simulink model "modelo"  (R2019b)
settings: Solver=ode45  StartTime=0.0  StopTime=0.5  MaxStep=1e-4  RelTol=1e-3
undefined symbols (not defined in the file or in its folder): GL, HL
settings Model: Creator=l54  LastModifiedBy=B13

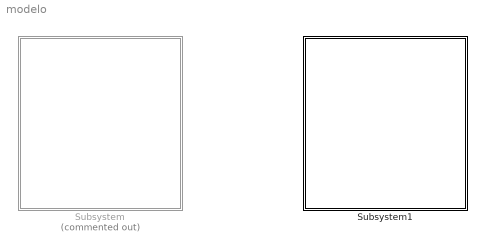
== system modelo ==
  Subsystem : Subsystem  Commented=on
  Subsystem1 : Subsystem

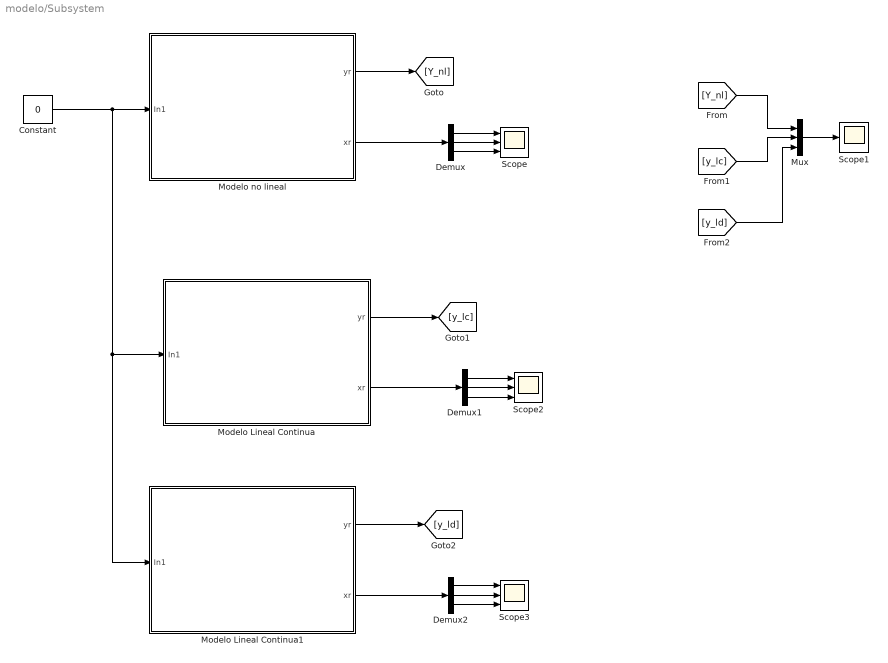
== system modelo/Subsystem ==
  Constant : Constant  Value=0
  Demux : Demux  Outputs=3
  Demux1 : Demux  Outputs=3
  Demux2 : Demux  Outputs=3
  Modelo Lineal Continua : Subsystem  mask(LEVITADOR MAGNETICO){g=9.81, M=0.05, R=10, L=0.5, xini=[0.01;0;0]}
      mask prompts: g "Gravedad"; M "Masa"; R "Resistencia"; L "Inductancia"; xini "Condiciones Iniciales"
      mask help: MODELO NO LINEAL DE UN LEVITADOR MAGENTICO
      mask init:
      | x10 = 0.16;
      | x20 = 0;
      | x30 = sqrt(g*M*x10);
      | AL = [0, 1, 0;
      |     x30^2/(M*x10^2), 0, -2*x30/(M*x10);
      |     0, 0, -R/L];
      | BL = [0;
      |     0;
      |     1/L];
      | CL = [1 0 0];
      | DL = 0;
      | eo = R*x30;
  Modelo Lineal Continua1 : Subsystem  mask(LEVITADOR MAGNETICO){g=9.81, M=0.05, R=10, L=0.5, xini=[0.01;0;0], Tm=0.01}
      mask prompts: g "Gravedad"; M "Masa"; R "Resistencia"; L "Inductancia"; xini "Condiciones Iniciales"; Tm "Periodo de muestreo"
      mask help: MODELO NO LINEAL DE UN LEVITADOR MAGENTICO
      mask init:
      | x10 = 0.16;
      | x20 = 0;
      | x30 = sqrt(g*M*x10);
      | AL = [0, 1, 0;
      |     x30^2/(M*x10^2), 0, -2*x30/(M*x10);
      |     0, 0, -R/L];
      | BL = [0;
      |     0;
      |     1/L];
      | CL = [1 0 0];
      | DL = 0;
      | eo = R*x30;
      | [GL,HL] = c2d(AL,BL,Tm);
  Modelo no lineal : Subsystem  mask(LEVITADOR MAGNETICO){g=9.81, M=0.05, R=10, L=0.5, xini=[0.01;0;0]}
      mask prompts: g "Gravedad"; M "Masa"; R "Resistencia"; L "Inductancia"; xini "Condiciones Iniciales"
      mask help: MODELO NO LINEAL DE UN LEVITADOR MAGENTICO
      mask init:
      | x10 = 0.16;
      | x20 = 0;
      | x30 = sqrt(g*M*x10);
      | CL = [1 0 0];
      | DL = 0;
      | eo = R*x30;
  Mux : Mux  Inputs=3
  Scope : Scope  NumInputPorts=3
  Scope1 : Scope
  Scope2 : Scope  NumInputPorts=3
  Scope3 : Scope  NumInputPorts=3
  wires:
  Demux2/3 -> Scope3/3
  [y_ld] -> Mux/3
  Constant/1 -> Modelo Lineal Continua1/1(In1), Modelo Lineal Continua/1(In1), Modelo no lineal/1(In1)
  Mux/1 -> Scope1/1
  Modelo no lineal/1(yr) -> [Y_nl]
  Demux1/3 -> Scope2/3
  Demux2/2 -> Scope3/2
  Demux/3 -> Scope/3
  Demux1/2 -> Scope2/2
  [Y_nl] -> Mux/1
  Demux1/1 -> Scope2/1
  Modelo Lineal Continua1/2(xr) -> Demux2/1
  Modelo Lineal Continua/2(xr) -> Demux1/1
  [y_lc] -> Mux/2
  Demux/2 -> Scope/2
  Modelo Lineal Continua1/1(yr) -> [y_ld]
  Demux/1 -> Scope/1
  Modelo Lineal Continua/1(yr) -> [y_lc]
  Demux2/1 -> Scope3/1
  Modelo no lineal/2(xr) -> Demux/1

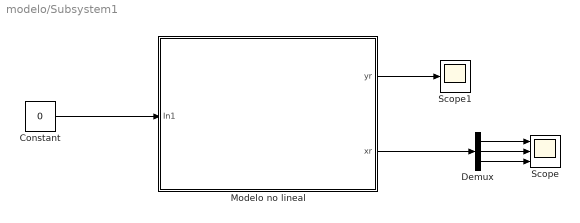
== system modelo/Subsystem1 ==
  Constant : Constant  Value=0
  Demux : Demux  Outputs=3
  Modelo no lineal : Subsystem  mask(LEVITADOR MAGNETICO){g=9.81, M=0.05, R=10, L=0.5, xini=[0;0;0]}
      mask prompts: g "Gravedad"; M "Masa"; R "Resistencia"; L "Inductancia"; xini "Condiciones Iniciales"
      mask help: MODELO NO LINEAL DE UN LEVITADOR MAGENTICO
      mask init:
      | x10 = 0.16;
      | x20 = 0;
      | x30 = sqrt(g*M*x10);
      | CL = [1 0 0];
      | DL = 0;
      | eo = R*x30;
  Scope : Scope  NumInputPorts=3
  Scope1 : Scope
  wires:
  Constant/1 -> Modelo no lineal/1(In1)
  Modelo no lineal/1(yr) -> Scope1/1
  Demux/3 -> Scope/3
  Demux/2 -> Scope/2
  Demux/1 -> Scope/1
  Modelo no lineal/2(xr) -> Demux/1

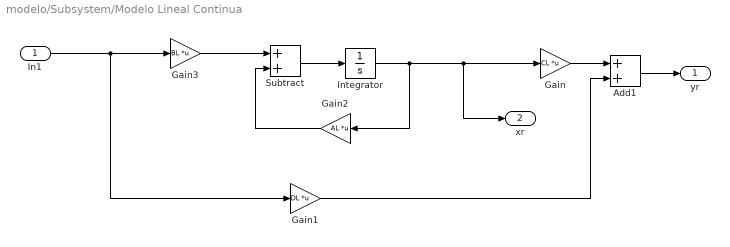
== system modelo/Subsystem/Modelo Lineal Continua ==
  In1 : Inport
  Add1 : Sum
  Gain : Gain  Gain=CL  Multiplication=Matrix(K*u)
  Gain1 : Gain  Gain=DL  Multiplication=Matrix(K*u)
  Gain2 : Gain  Gain=AL  Multiplication=Matrix(K*u)
  Gain3 : Gain  Gain=BL  Multiplication=Matrix(K*u)
  Integrator : Integrator  InitialCondition=xini
  Subtract : Sum
  yr : Outport
  xr : Outport  Port=2
  wires:
  In1/1 -> Gain3/1, Gain1/1
  Integrator/1 -> Gain/1, xr/1, Gain2/1
  Add1/1 -> yr/1
  Gain/1 -> Add1/1
  Gain1/1 -> Add1/2
  Subtract/1 -> Integrator/1
  Gain2/1 -> Subtract/2
  Gain3/1 -> Subtract/1

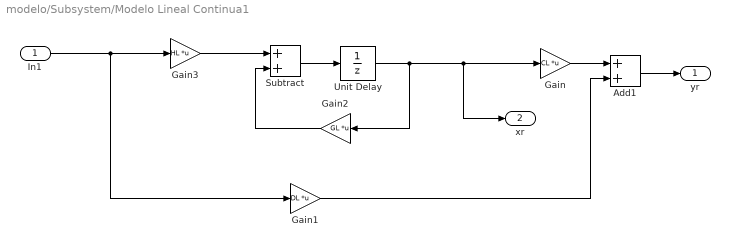
== system modelo/Subsystem/Modelo Lineal Continua1 ==
  In1 : Inport
  Add1 : Sum
  Gain : Gain  Gain=CL  Multiplication=Matrix(K*u)
  Gain1 : Gain  Gain=DL  Multiplication=Matrix(K*u)
  Gain2 : Gain  Gain=GL  Multiplication=Matrix(K*u)
  Gain3 : Gain  Gain=HL  Multiplication=Matrix(K*u)
  Subtract : Sum
  Unit Delay : UnitDelay  InitialCondition=xini  SampleTime=Tm  HasFrameUpgradeWarning=on
  yr : Outport
  xr : Outport  Port=2
  wires:
  In1/1 -> Gain3/1, Gain1/1
  Unit Delay/1 -> Gain/1, xr/1, Gain2/1
  Add1/1 -> yr/1
  Gain/1 -> Add1/1
  Gain1/1 -> Add1/2
  Subtract/1 -> Unit Delay/1
  Gain2/1 -> Subtract/2
  Gain3/1 -> Subtract/1

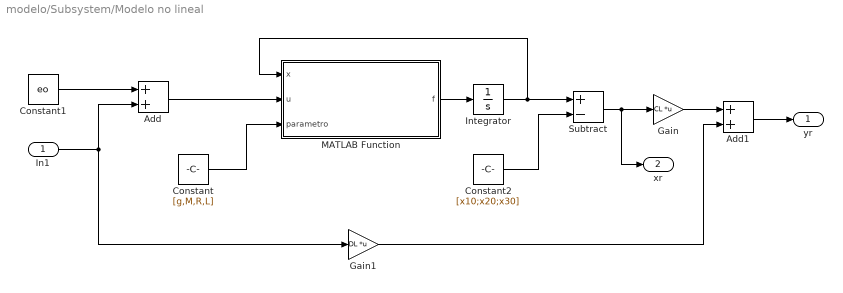
== system modelo/Subsystem/Modelo no lineal ==
  In1 : Inport
  Add : Sum
  Add1 : Sum
  Constant : Constant  Value=[g,M,R,L]
  Constant1 : Constant  Value=eo
  Constant2 : Constant  Value=[x10;x20;x30]
  Gain : Gain  Gain=CL  Multiplication=Matrix(K*u)
  Gain1 : Gain  Gain=DL  Multiplication=Matrix(K*u)
  Integrator : Integrator  InitialCondition=[x10; x20; x30]+xini
  MATLAB Function : MATLAB Function  TreatAsAtomicUnit=on
  Subtract : Sum  Inputs=+-
  yr : Outport
  xr : Outport  Port=2
  wires:
  Integrator/1 -> MATLAB Function/1(x), Subtract/1
  In1/1 -> Gain1/1, Add/2
  MATLAB Function/1(f) -> Integrator/1
  Add/1 -> MATLAB Function/2(u)
  Constant1/1 -> Add/1
  Subtract/1 -> xr/1, Gain/1
  Constant2/1 -> Subtract/2
  Constant/1 -> MATLAB Function/3(parametro)
  Add1/1 -> yr/1
  Gain/1 -> Add1/1
  Gain1/1 -> Add1/2

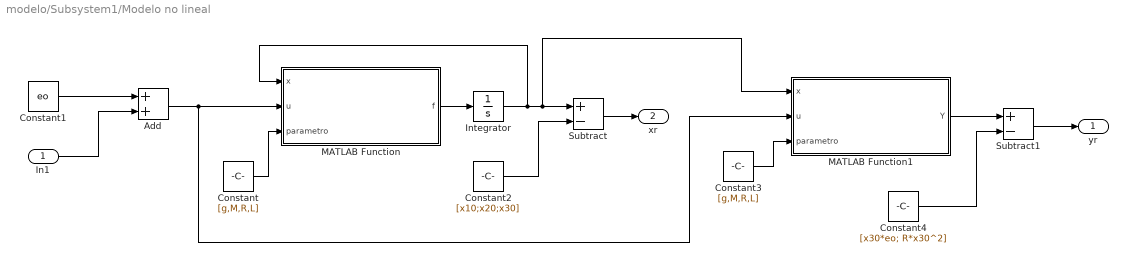
== system modelo/Subsystem1/Modelo no lineal ==
  In1 : Inport
  Add : Sum
  Constant : Constant  Value=[g,M,R,L]
  Constant1 : Constant  Value=eo
  Constant2 : Constant  Value=[x10;x20;x30]
  Constant3 : Constant  Value=[g,M,R,L]
  Constant4 : Constant  Value=[x30*eo; R*x30^2]
  Integrator : Integrator  InitialCondition=[x10; x20; x30]+xini
  MATLAB Function : MATLAB Function  TreatAsAtomicUnit=on
  MATLAB Function1 : MATLAB Function  TreatAsAtomicUnit=on
  Subtract : Sum  Inputs=+-
  Subtract1 : Sum  Inputs=+-
  yr : Outport
  xr : Outport  Port=2
  wires:
  Integrator/1 -> MATLAB Function/1(x), MATLAB Function1/1(x), Subtract/1
  In1/1 -> Add/2
  MATLAB Function/1(f) -> Integrator/1
  Add/1 -> MATLAB Function/2(u), MATLAB Function1/2(u)
  Constant1/1 -> Add/1
  Subtract/1 -> xr/1
  Constant2/1 -> Subtract/2
  Constant/1 -> MATLAB Function/3(parametro)
  Constant3/1 -> MATLAB Function1/3(parametro)
  MATLAB Function1/1(Y) -> Subtract1/1
  Constant4/1 -> Subtract1/2
  Subtract1/1 -> yr/1

== matlab function modelo/Subsystem1/Modelo no lineal/MATLAB Function ==
  data: x input; u input; f output; parametro input
function f = fcn(x,u,parametro)
x1 = x(1);
x2 = x(2);
x3 = x(3);
e = u;
g = parametro(1);
M = parametro(2);
R = parametro(3);
L = parametro(4);
f1 = x2;
f2 = g - x3^2/(M*x1);
f3 = -R*x3/L + e/L;
f = [f1;f2;f3];

== matlab function modelo/Subsystem/Modelo no lineal/MATLAB Function ==
  data: x input; u input; f output; parametro input
function f = fcn(x,u,parametro)
x1 = x(1);
x2 = x(2);
x3 = x(3);
e = u;
g = parametro(1);
M = parametro(2);
R = parametro(3);
L = parametro(4);
f1 = x2;
f2 = g - x3^2/(M*x1);
f3 = -R*x3/L + e/L;
f = [f1;f2;f3];

== matlab function modelo/Subsystem1/Modelo no lineal/MATLAB Function1 ==
  data: x input; u input; Y output; parametro input
function Y = fcn(x,u,parametro)
x1 = x(1);
x2 = x(2);
x3 = x(3);
e = u;
g = parametro(1);
M = parametro(2);
R = parametro(3);
L = parametro(4);
y1 = e*x3;
y2 = R*x3^2;
Y = [y1;y2];
